simulink model "vectorResizer"  (R2022b)
settings: Solver=FixedStepAuto  StartTime=0.0  StopTime=291  FixedStep=1  RelTol=1e-3
values from neighbouring files (symbols this model uses):
  cyc_mph = cell2mat(struct2cell(load(strcat(folder_name,driving_cycle_name,'_cyc_mph'))))    [graficiFinali.m]
  PredictionHorizon = 10    [main.m]
undefined symbols (not defined in the file or in its folder): eta_DC_AC, eta_drive, eta_EM, veh_air_density, veh_CD, veh_FA, veh_gravity, veh_mass, wh_1st_rrc
libraries: simulink x1
settings Model: Creator=William  LastModifiedBy=William

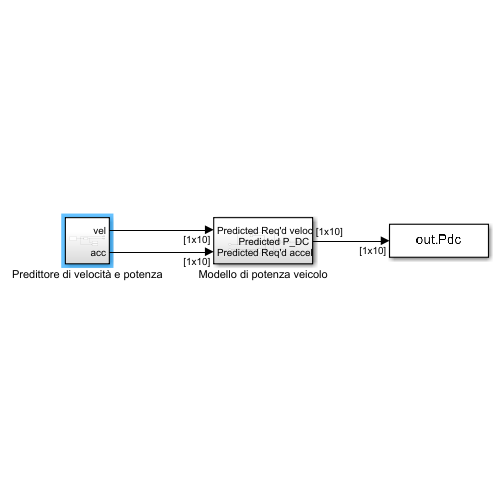
[thumbnail: Simulink's stored preview of the top-level diagram]
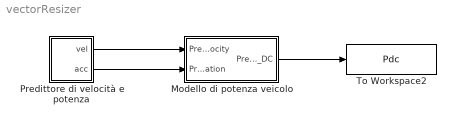
== system vectorResizer ==
  Modello di potenza veicolo : Subsystem
  Predittore di velocità e potenza : Subsystem
  To Workspace2 : ToWorkspace  VariableName=Pdc  SaveFormat=Structure  SampleTime=-1
  wires:
  Modello di potenza veicolo/1(Predicted P_DC) -> To Workspace2/1
  Predittore di velocità e potenza/1(vel) -> Modello di potenza veicolo/1(Predicted Req'd velocity)
  Predittore di velocità e potenza/2(acc) -> Modello di potenza veicolo/2(Predicted Req'd acceleration)

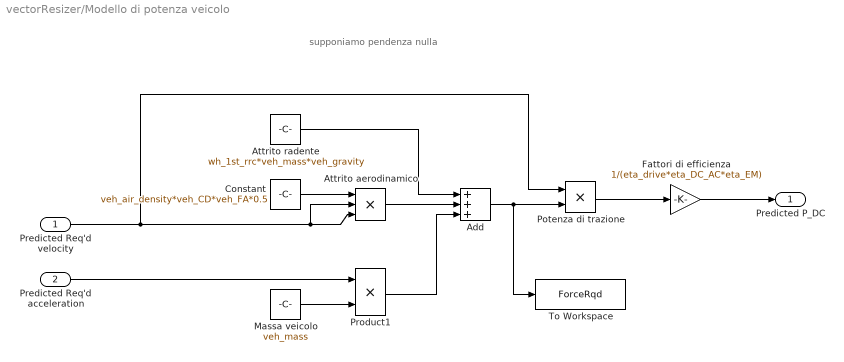
== system vectorResizer/Modello di potenza veicolo ==
  note: supponiamo pendenza nulla
  Predicted Req'd velocity : Inport
  Predicted Req'd acceleration : Inport  Port=2
  Add : Sum  Inputs=+++
  Attrito aerodinamico : Product  Inputs=3
  Attrito radente : Constant  Value=wh_1st_rrc*veh_mass*veh_gravity
  Constant : Constant  Value=veh_air_density*veh_CD*veh_FA*0.5
  Fattori di efficienza : Gain  Gain=1/(eta_drive*eta_DC_AC*eta_EM)
  Massa veicolo : Constant  Value=veh_mass
  Potenza di trazione : Product
  Product1 : Product
  To Workspace : ToWorkspace  VariableName=ForceRqd  SaveFormat=Structure  SampleTime=-1
  Predicted P_DC : Outport
  wires:
  Product1/1 -> Add/3
  Attrito aerodinamico/1 -> Add/2
  Add/1 -> To Workspace/1, Potenza di trazione/2
  Potenza di trazione/1 -> Fattori di efficienza/1
  Attrito radente/1 -> Add/1
  Predicted Req'd velocity/1 -> Potenza di trazione/1, Attrito aerodinamico/3, Attrito aerodinamico/2
  Constant/1 -> Attrito aerodinamico/1
  Fattori di efficienza/1 -> Predicted P_DC/1
  Massa veicolo/1 -> Product1/2
  Predicted Req'd acceleration/1 -> Product1/1

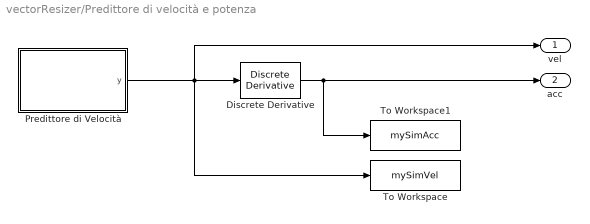
== system vectorResizer/Predittore di velocità e potenza ==
  Discrete Derivative : simulink/Discrete/Discrete Derivative  gainval=1.0  ICPrevScaledInput=0.0  OutMin=[]  OutMax=[]  OutDataType=fixdt(1, 16)  OutScaling=2^-10  DoSatur=off
  Predittore di Velocità : Subsystem
  To Workspace : ToWorkspace  VariableName=mySimVel  SaveFormat=Structure  SampleTime=-1
  To Workspace1 : ToWorkspace  VariableName=mySimAcc  SaveFormat=Structure  SampleTime=-1
  vel : Outport
  acc : Outport  Port=2
  wires:
  Discrete Derivative/1 -> acc/1, To Workspace1/1
  Predittore di Velocità/1(y) -> vel/1, Discrete Derivative/1, To Workspace/1

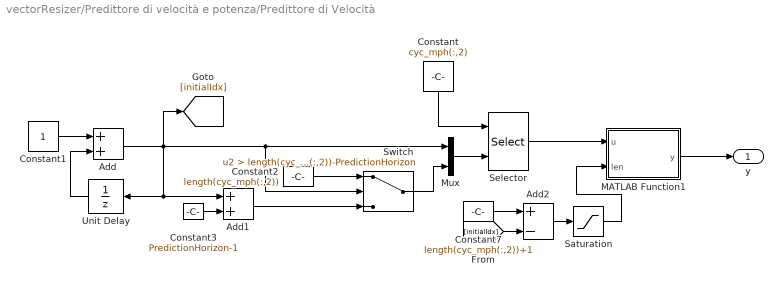
== system vectorResizer/Predittore di velocità e potenza/Predittore di Velocità ==
  Add : Sum
  Add1 : Sum
  Add2 : Sum  Inputs=+-
  Constant : Constant  Value=cyc_mph(:,2)  VectorParams1D=off
  Constant1 : Constant
  Constant2 : Constant  Value=length(cyc_mph(:,2))
  Constant3 : Constant  Value=PredictionHorizon-1
  Constant7 : Constant  Value=length(cyc_mph(:,2))+1
  MATLAB Function1 : MATLAB Function  TreatAsAtomicUnit=on
  Mux : Mux  Inputs=2
  Saturation : Saturate  UpperLimit=10
  Selector : Selector  IndexOptions=Starting and ending indices (port)  Indices=[1 3]  OutputSizes=10
  Switch : Switch  Criteria=u2 > Threshold  Threshold=length(cyc_mph(:,2))-PredictionHorizon  SaturateOnIntegerOverflow=off  InputSameDT=off
  Unit Delay : UnitDelay  SampleTime=-1  HasFrameUpgradeWarning=on
  y : Outport
  wires:
  Mux/1 -> Selector/2
  Constant/1 -> Selector/1
  [initialIdx] -> Add2/2
  Constant1/1 -> Add/1
  Add2/1 -> Saturation/1
  Constant3/1 -> Add1/2
  Unit Delay/1 -> Add/2
  Switch/1 -> Mux/2
  Selector/1 -> MATLAB Function1/1(u)
  Constant7/1 -> Add2/1
  Constant2/1 -> Switch/1
  Add1/1 -> Switch/3
  Add/1 -> [initialIdx], Unit Delay/1, Add1/1, Switch/2, Mux/1
  Saturation/1 -> MATLAB Function1/2(len)
  MATLAB Function1/1(y) -> y/1

== matlab function vectorResizer/Predittore di velocità e potenza/Predittore di Velocità/MATLAB Function1 ==
  data: u input; y output size=[1 10]; len input
function y = fcn(u,len)

y = zeros(1,10);
y(1:len) = u(1:len)';

if len<10
    y(len:10)=u(len);
end
